simulink model "RoboticArmController"  (R2022b)
settings: Solver=FixedStepAuto  StartTime=0.0  StopTime=10.0  FixedStep=1  RelTol=1e-3
libraries: simulink x50
(part 2 of 2)

== system RoboticArmController/Main/Start/Handle/FindInPool/FindArmIdInPool ==
  ArmId : Inport
  AND : Logic  IconShape=distinctive  AllPortsSameDT=off  OutDataTypeStr=boolean
  Compare To Constant : simulink/Logic and Bit Operations/Compare To Constant  relop===  const=1  OutDataTypeStr=boolean
  Constant : Constant  OutDataTypeStr=boolean
  Data Store Read : DataStoreRead  DataStoreName=ArmIdPool  IndexOptions=Index vector (dialog)  Indices=1  OutputSizes=1
  Data Store Read1 : DataStoreRead  DataStoreName=Found  IndexOptions=Index vector (dialog)  Indices=1  OutputSizes=1
  Data Store Read2 : DataStoreRead  DataStoreName=ArmIdPoolF  IndexOptions=Index vector (dialog)  Indices=1  OutputSizes=1
  Data Store Write1 : DataStoreWrite  DataStoreName=Found  IndexOptions=Index vector (dialog)  Indices=1  OutputSizes=1
  Equal : RelationalOperator  Operator===  OutDataTypeStr=boolean  RndMeth=Simplest  InputSameDT=off
  For Iterator : ForIterator  IterationLimit=POOL_SIZE  IndexMode=Zero-based
  Selector : Selector  IndexMode=Zero-based  InputPortWidth=POOL_SIZE  IndexOptions=Index vector (port)  Indices=[1 3]  OutputSizes=1
  Selector1 : Selector  IndexMode=Zero-based  InputPortWidth=POOL_SIZE  IndexOptions=Index vector (port)  Indices=[1 3]  OutputSizes=1
  Switch : Switch  Criteria=u2 ~= 0  SaturateOnIntegerOverflow=off  InputSameDT=off
  Out1 : Outport
  wires:
  For Iterator/1 -> Selector1/2, Selector/2
  Data Store Read/1 -> Selector/1
  Selector/1 -> Equal/1
  ArmId/1 -> Equal/2
  Equal/1 -> AND/1
  Constant/1 -> Switch/1
  Switch/1 -> Out1/1, Data Store Write1/1
  Data Store Read1/1 -> Switch/3
  Data Store Read2/1 -> Selector1/1
  Selector1/1 -> Compare To Constant/1
  Compare To Constant/1 -> AND/2
  AND/1 -> Switch/2

== system RoboticArmController/Main/Start/Handle/FindInPool/FindEmptyInPool ==
  AND : Logic  IconShape=distinctive  AllPortsSameDT=off  OutDataTypeStr=boolean
  Compare To Constant1 : simulink/Logic and Bit Operations/Compare To Constant  relop===  const=-1  OutDataTypeStr=boolean
  Compare To Constant2 : simulink/Logic and Bit Operations/Compare To Constant  relop===  const=0  OutDataTypeStr=boolean
  Data Store Read1 : DataStoreRead  DataStoreName=Found_E  IndexOptions=Index vector (dialog)  Indices=1  OutputSizes=1
  Data Store Read2 : DataStoreRead  DataStoreName=ArmIdPoolF  IndexOptions=Index vector (dialog)  Indices=1  OutputSizes=1
  Data Store Write1 : DataStoreWrite  DataStoreName=Found_E  IndexOptions=Index vector (dialog)  Indices=1  OutputSizes=1
  For Iterator : ForIterator  IterationLimit=POOL_SIZE  IndexMode=Zero-based
  Selector1 : Selector  IndexMode=Zero-based  InputPortWidth=POOL_SIZE  IndexOptions=Index vector (port)  Indices=[1 3]  OutputSizes=1
  Switch : Switch  Criteria=u2 ~= 0  SaturateOnIntegerOverflow=off  InputSameDT=off
  Out1 : Outport
  wires:
  Switch/1 -> Data Store Write1/1, Out1/1
  Data Store Read1/1 -> Compare To Constant1/1, Switch/3
  Compare To Constant1/1 -> AND/2
  AND/1 -> Switch/2
  For Iterator/1 -> Selector1/2, Switch/1
  Selector1/1 -> Compare To Constant2/1
  Data Store Read2/1 -> Selector1/1
  Compare To Constant2/1 -> AND/1

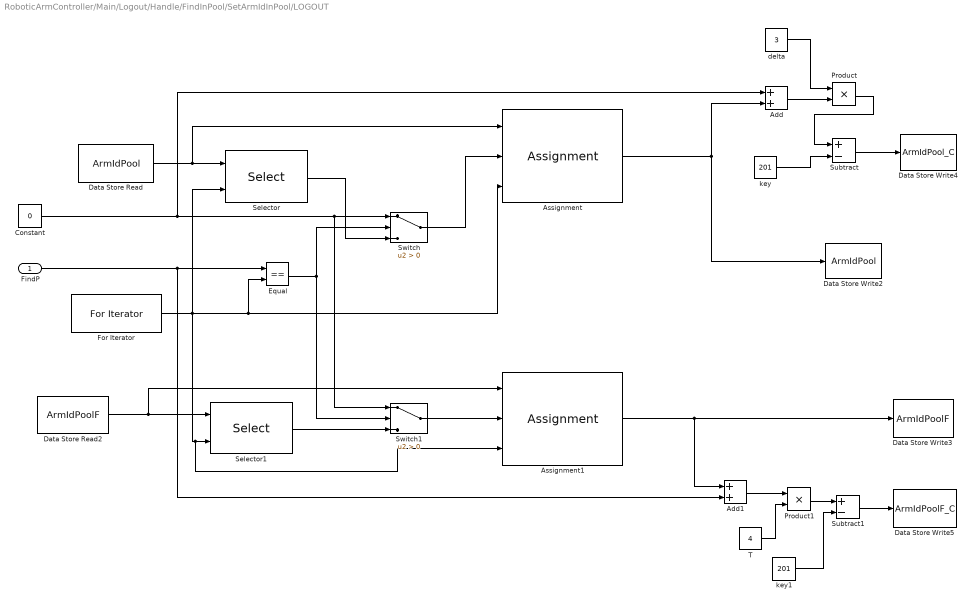
== system RoboticArmController/Main/Logout/Handle/FindInPool/SetArmIdInPool/LOGOUT ==
  FindP : Inport
  Add : Sum  OutDataTypeStr=int32
  Add1 : Sum  OutDataTypeStr=int32
  Assignment : Assignment  IndexMode=Zero-based  DiagnosticForDimensions=Warning  IndexOptions=Index vector (port)  Indices=1  OutputSizes=1
  Assignment1 : Assignment  IndexMode=Zero-based  DiagnosticForDimensions=Warning  IndexOptions=Index vector (port)  Indices=1  OutputSizes=1
  Constant : Constant  Value=0  OutDataTypeStr=int32
  Data Store Read : DataStoreRead  DataStoreName=ArmIdPool  IndexOptions=Index vector (dialog)  Indices=1  OutputSizes=1
  Data Store Read2 : DataStoreRead  DataStoreName=ArmIdPoolF  IndexOptions=Index vector (dialog)  Indices=1  OutputSizes=1
  Data Store Write2 : DataStoreWrite  DataStoreName=ArmIdPool  IndexOptions=Index vector (dialog)  Indices=1  OutputSizes=1
  Data Store Write3 : DataStoreWrite  DataStoreName=ArmIdPoolF  IndexOptions=Index vector (dialog)  Indices=1  OutputSizes=1
  Data Store Write4 : DataStoreWrite  DataStoreName=ArmIdPool_C  IndexOptions=Index vector (dialog)  Indices=1  OutputSizes=1
  Data Store Write5 : DataStoreWrite  DataStoreName=ArmIdPoolF_C  IndexOptions=Index vector (dialog)  Indices=1  OutputSizes=1
  Equal : RelationalOperator  Operator===  OutDataTypeStr=boolean  RndMeth=Simplest  InputSameDT=off
  For Iterator : ForIterator  IterationLimit=POOL_SIZE  IndexMode=Zero-based
  Product : Product  OutDataTypeStr=int32
  Product1 : Product  OutDataTypeStr=int32
  Selector : Selector  IndexMode=Zero-based  InputPortWidth=POOL_SIZE  IndexOptions=Index vector (port)  Indices=[1 3]  OutputSizes=1
  Selector1 : Selector  IndexMode=Zero-based  InputPortWidth=POOL_SIZE  IndexOptions=Index vector (port)  Indices=[1 3]  OutputSizes=1
  Subtract : Sum  Inputs=+-  OutDataTypeStr=int32
  Subtract1 : Sum  Inputs=+-  OutDataTypeStr=int32
  Switch : Switch  Criteria=u2 > Threshold  SaturateOnIntegerOverflow=off  InputSameDT=off
  Switch1 : Switch  Criteria=u2 > Threshold  SaturateOnIntegerOverflow=off  InputSameDT=off
  T : Constant  Value=4  OutDataTypeStr=int32
  delta : Constant  Value=3  OutDataTypeStr=int32
  key : Constant  Value=201  OutDataTypeStr=int32
  key1 : Constant  Value=201  OutDataTypeStr=int32
  wires:
  For Iterator/1 -> Assignment1/3, Selector1/2, Selector/2, Assignment/3, Equal/2
  Data Store Read/1 -> Assignment/1, Selector/1
  FindP/1 -> Add1/2, Equal/1
  Equal/1 -> Switch/2, Switch1/2
  Switch/1 -> Assignment/2
  Selector/1 -> Switch/3
  Constant/1 -> Add/1, Switch1/1, Switch/1
  Data Store Read2/1 -> Assignment1/1, Selector1/1
  Selector1/1 -> Switch1/3
  Switch1/1 -> Assignment1/2
  Subtract/1 -> Data Store Write4/1
  key/1 -> Subtract/2
  T/1 -> Product1/2
  key1/1 -> Subtract1/2
  Assignment1/1 -> Add1/1, Data Store Write3/1
  Product1/1 -> Subtract1/1
  Assignment/1 -> Data Store Write2/1, Add/2
  Add1/1 -> Product1/1
  delta/1 -> Product/1
  Add/1 -> Product/2
  Product/1 -> Subtract/1
  Subtract1/1 -> Data Store Write5/1

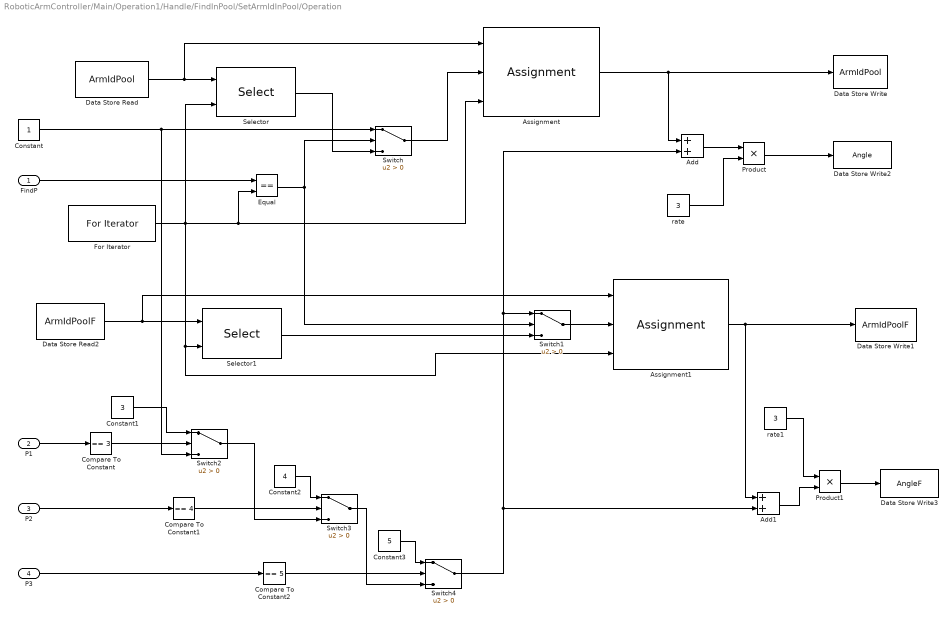
== system RoboticArmController/Main/Operation1/Handle/FindInPool/SetArmIdInPool/Operation ==
  FindP : Inport
  P1 : Inport  Port=2
  P2 : Inport  Port=3
  P3 : Inport  Port=4
  Add : Sum  AccumDataTypeStr=int32
  Add1 : Sum  AccumDataTypeStr=int32
  Assignment : Assignment  IndexMode=Zero-based  DiagnosticForDimensions=Warning  IndexOptions=Index vector (port)  Indices=1  OutputSizes=1
  Assignment1 : Assignment  IndexMode=Zero-based  DiagnosticForDimensions=Warning  IndexOptions=Index vector (port)  Indices=1  OutputSizes=1
  Compare To Constant : simulink/Logic and Bit Operations/Compare To Constant  relop===  const=3  OutDataTypeStr=boolean
  Compare To Constant1 : simulink/Logic and Bit Operations/Compare To Constant  relop===  const=4  OutDataTypeStr=boolean
  Compare To Constant2 : simulink/Logic and Bit Operations/Compare To Constant  relop===  const=5  OutDataTypeStr=boolean
  Constant : Constant  OutDataTypeStr=int32
  Constant1 : Constant  Value=3  OutDataTypeStr=int32
  Constant2 : Constant  Value=4  OutDataTypeStr=int32
  Constant3 : Constant  Value=5  OutDataTypeStr=int32
  Data Store Read : DataStoreRead  DataStoreName=ArmIdPool  IndexOptions=Index vector (dialog)  Indices=1  OutputSizes=1
  Data Store Read2 : DataStoreRead  DataStoreName=ArmIdPoolF  IndexOptions=Index vector (dialog)  Indices=1  OutputSizes=1
  Data Store Write : DataStoreWrite  DataStoreName=ArmIdPool  IndexOptions=Index vector (dialog)  Indices=1  OutputSizes=1
  Data Store Write1 : DataStoreWrite  DataStoreName=ArmIdPoolF  IndexOptions=Index vector (dialog)  Indices=1  OutputSizes=1
  Data Store Write2 : DataStoreWrite  DataStoreName=Angle  IndexOptions=Index vector (dialog)  Indices=1  OutputSizes=1
  Data Store Write3 : DataStoreWrite  DataStoreName=AngleF  IndexOptions=Index vector (dialog)  Indices=1  OutputSizes=1
  Equal : RelationalOperator  Operator===  OutDataTypeStr=boolean  RndMeth=Simplest  InputSameDT=off
  For Iterator : ForIterator  IterationLimit=POOL_SIZE  IndexMode=Zero-based
  Product : Product  OutDataTypeStr=int32
  Product1 : Product  OutDataTypeStr=int32
  Selector : Selector  IndexMode=Zero-based  InputPortWidth=POOL_SIZE  IndexOptions=Index vector (port)  Indices=[1 3]  OutputSizes=1
  Selector1 : Selector  IndexMode=Zero-based  InputPortWidth=POOL_SIZE  IndexOptions=Index vector (port)  Indices=[1 3]  OutputSizes=1
  Switch{,1..4} (5 alike) : Switch  Criteria=u2 > Threshold  SaturateOnIntegerOverflow=off  InputSameDT=off
  rate : Constant  Value=3
  rate1 : Constant  Value=3
  wires:
  For Iterator/1 -> Selector1/2, Assignment1/3, Selector/2, Assignment/3, Equal/2
  Data Store Read/1 -> Assignment/1, Selector/1
  FindP/1 -> Equal/1
  Equal/1 -> Switch/2, Switch1/2
  Switch/1 -> Assignment/2
  Selector/1 -> Switch/3
  Assignment/1 -> Add/1, Data Store Write/1
  Constant/1 -> Switch2/3, Switch/1
  Data Store Read2/1 -> Assignment1/1, Selector1/1
  Selector1/1 -> Switch1/3
  Assignment1/1 -> Data Store Write1/1, Add1/1
  Switch1/1 -> Assignment1/2
  P1/1 -> Compare To Constant/1
  Constant1/1 -> Switch2/1
  Compare To Constant/1 -> Switch2/2
  Switch2/1 -> Switch3/3
  Compare To Constant1/1 -> Switch3/2
  Constant2/1 -> Switch3/1
  P2/1 -> Compare To Constant1/1
  Compare To Constant2/1 -> Switch4/2
  P3/1 -> Compare To Constant2/1
  Switch4/1 -> Add/2, Switch1/1, Add1/2
  Switch3/1 -> Switch4/3
  Constant3/1 -> Switch4/1
  Add/1 -> Product/1
  Product/1 -> Data Store Write2/1
  rate/1 -> Product/2
  Add1/1 -> Product1/2
  rate1/1 -> Product1/1
  Product1/1 -> Data Store Write3/1

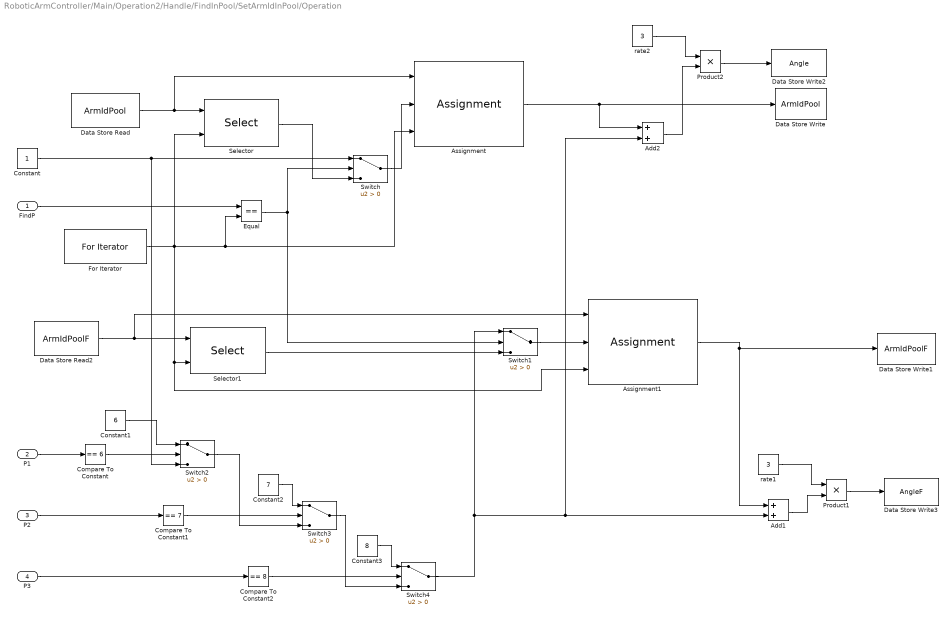
== system RoboticArmController/Main/Operation2/Handle/FindInPool/SetArmIdInPool/Operation ==
  FindP : Inport
  P1 : Inport  Port=2
  P2 : Inport  Port=3
  P3 : Inport  Port=4
  Add1 : Sum  AccumDataTypeStr=int32
  Add2 : Sum  AccumDataTypeStr=int32
  Assignment : Assignment  IndexMode=Zero-based  DiagnosticForDimensions=Warning  IndexOptions=Index vector (port)  Indices=1  OutputSizes=1
  Assignment1 : Assignment  IndexMode=Zero-based  DiagnosticForDimensions=Warning  IndexOptions=Index vector (port)  Indices=1  OutputSizes=1
  Compare To Constant : simulink/Logic and Bit Operations/Compare To Constant  relop===  const=6  OutDataTypeStr=boolean
  Compare To Constant1 : simulink/Logic and Bit Operations/Compare To Constant  relop===  const=7  OutDataTypeStr=boolean
  Compare To Constant2 : simulink/Logic and Bit Operations/Compare To Constant  relop===  const=8  OutDataTypeStr=boolean
  Constant : Constant  OutDataTypeStr=int32
  Constant1 : Constant  Value=6  OutDataTypeStr=int32
  Constant2 : Constant  Value=7  OutDataTypeStr=int32
  Constant3 : Constant  Value=8  OutDataTypeStr=int32
  Data Store Read : DataStoreRead  DataStoreName=ArmIdPool  IndexOptions=Index vector (dialog)  Indices=1  OutputSizes=1
  Data Store Read2 : DataStoreRead  DataStoreName=ArmIdPoolF  IndexOptions=Index vector (dialog)  Indices=1  OutputSizes=1
  Data Store Write : DataStoreWrite  DataStoreName=ArmIdPool  IndexOptions=Index vector (dialog)  Indices=1  OutputSizes=1
  Data Store Write1 : DataStoreWrite  DataStoreName=ArmIdPoolF  IndexOptions=Index vector (dialog)  Indices=1  OutputSizes=1
  Data Store Write2 : DataStoreWrite  DataStoreName=Angle  IndexOptions=Index vector (dialog)  Indices=1  OutputSizes=1
  Data Store Write3 : DataStoreWrite  DataStoreName=AngleF  IndexOptions=Index vector (dialog)  Indices=1  OutputSizes=1
  Equal : RelationalOperator  Operator===  OutDataTypeStr=boolean  RndMeth=Simplest  InputSameDT=off
  For Iterator : ForIterator  IterationLimit=POOL_SIZE  IndexMode=Zero-based
  Product1 : Product  OutDataTypeStr=int32
  Product2 : Product  OutDataTypeStr=int32
  Selector : Selector  IndexMode=Zero-based  InputPortWidth=POOL_SIZE  IndexOptions=Index vector (port)  Indices=[1 3]  OutputSizes=1
  Selector1 : Selector  IndexMode=Zero-based  InputPortWidth=POOL_SIZE  IndexOptions=Index vector (port)  Indices=[1 3]  OutputSizes=1
  Switch{,1..4} (5 alike) : Switch  Criteria=u2 > Threshold  SaturateOnIntegerOverflow=off  InputSameDT=off
  rate1 : Constant  Value=3
  rate2 : Constant  Value=3
  wires:
  For Iterator/1 -> Selector1/2, Assignment1/3, Selector/2, Assignment/3, Equal/2
  Data Store Read/1 -> Assignment/1, Selector/1
  FindP/1 -> Equal/1
  Equal/1 -> Switch/2, Switch1/2
  Switch/1 -> Assignment/2
  Selector/1 -> Switch/3
  Assignment/1 -> Add2/1, Data Store Write/1
  Constant/1 -> Switch2/3, Switch/1
  Data Store Read2/1 -> Assignment1/1, Selector1/1
  Selector1/1 -> Switch1/3
  Assignment1/1 -> Add1/1, Data Store Write1/1
  Switch1/1 -> Assignment1/2
  P1/1 -> Compare To Constant/1
  Constant1/1 -> Switch2/1
  Compare To Constant/1 -> Switch2/2
  Switch2/1 -> Switch3/3
  Compare To Constant1/1 -> Switch3/2
  Constant2/1 -> Switch3/1
  P2/1 -> Compare To Constant1/1
  Compare To Constant2/1 -> Switch4/2
  P3/1 -> Compare To Constant2/1
  Switch4/1 -> Switch1/1, Add2/2, Add1/2
  Switch3/1 -> Switch4/3
  Constant3/1 -> Switch4/1
  rate1/1 -> Product1/1
  Add1/1 -> Product1/2
  Product1/1 -> Data Store Write3/1
  Product2/1 -> Data Store Write2/1
  Add2/1 -> Product2/2
  rate2/1 -> Product2/1
